simulink model "camera_only"  (R2016a)
settings: Solver=ode45  StartTime=0.0  StopTime=inf  FixedStep=0.005  RelTol=1e-3
InitFcn:
  | param
undefined symbols (not defined in the file or in its folder): camera, drawCamera, P, velocity_command
settings Model: Creator=magiccjae  LastModifiedBy=magiccjae

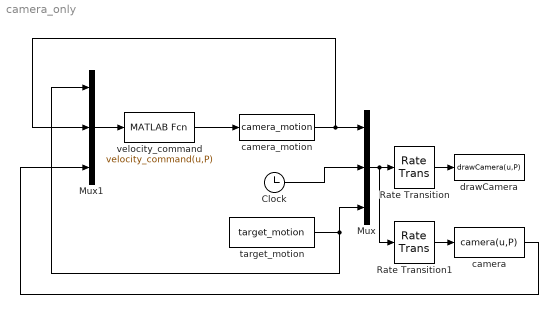
== system camera_only ==
  Clock : Clock
  Mux : Mux  Inputs=3
  Mux1 : Mux  Inputs=3
  Rate Transition : RateTransition  OutPortSampleTime=[0.05,0]
  Rate Transition1 : RateTransition  OutPortSampleTime=[0.02,0]
  camera : MATLABFcn  MATLABFcn=camera(u,P)
  camera_motion : S-Function  FunctionName=camera_motion  Parameters=P  SFunctionDeploymentMode=off  EnableBusSupport=off
  drawCamera : MATLABFcn  MATLABFcn=drawCamera(u,P)  OutputDimensions=0
  target_motion : S-Function  FunctionName=target_motion  Parameters=P  SFunctionDeploymentMode=off  EnableBusSupport=off
  velocity_command : MATLABFcn  MATLABFcn=velocity_command(u,P)  OutputDimensions=6
  wires:
  camera_motion/1 -> Mux1/2, Mux/1
  velocity_command/1 -> camera_motion/1
  Clock/1 -> Mux/2
  Mux/1 -> Rate Transition1/1, Rate Transition/1
  Rate Transition/1 -> drawCamera/1
  target_motion/1 -> Mux1/1, Mux/3
  Mux1/1 -> velocity_command/1
  camera/1 -> Mux1/3
  Rate Transition1/1 -> camera/1
